simulink model "UnTrans_sim1"  (R2015a)
settings: Solver=ode3  StartTime=0.0  StopTime=10.0  FixedStep=0.01  RelTol=1e-3
undefined symbols (not defined in the file or in its folder): NL
settings Model: CovSFcnEnable=off  Creator=kha  LastModifiedBy=RBoth
settings DataIOCC: SignalLoggingSaveFormat=ModelDataLogs
settings OptimizationCC: ExpressionDepthLimit=2147483647
settings DebuggingCC: UnderspecifiedInitializationDetection=Classic  MergeDetectMultiDrivingBlocksExec=none  SolverPrmCheckMsg=warning  FcnCallInpInsideContextMsg=EnableAllAsWarning  StateNameClashWarn=warning
settings GRTTargetCC: CombineOutputUpdateFcns=off  GRTInterface=on

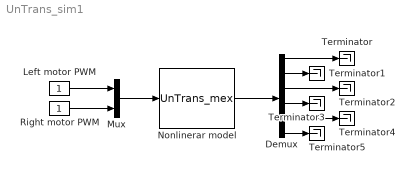
== system UnTrans_sim1 ==
  Demux : Demux  Outputs=6
  Left motor PWM : Constant
  Mux : Mux  Inputs=2
  Nonlinerar model : S-Function  InitFcn=|  FunctionName=UnTrans_mex  Parameters=x0, [NL.d1, NL.d2, NL.c1, NL.c2, NL.c3, NL.Jd, NL.MRL, NL.MLL, NL.MgL, NL.W2R, NL.Ffw]  mask(S-function: untrans){x0=[0 0 0.1 0 0 0], NL=NL}
      | UnTransPar = UnTransParams( );           
      | [NL] = UnTransNonlinearModel(UnTransPar);
      mask prompts: x0 "Initial conditions: [theta, theta',psi,psi',phi,phi']"; NL "Model Parameters"
      mask help:
      | This is a S-function block which implements
      | nonlinear model of two wheeled balancing robot.
      mask Display: image( imread('Trans_non.jpg','jpg') )
  Right motor PWM : Constant
  Terminator{,1..5} (6 alike) : Terminator
  wires:
  Mux/1 -> Nonlinerar model/1
  Nonlinerar model/1 -> Demux/1
  Left motor PWM/1 -> Mux/1
  Right motor PWM/1 -> Mux/2
  Demux/1 -> Terminator/1
  Demux/2 -> Terminator1/1
  Demux/3 -> Terminator2/1
  Demux/4 -> Terminator3/1
  Demux/5 -> Terminator4/1
  Demux/6 -> Terminator5/1
